simulink model "Problema_2_simulink_f"  (R2014a)
settings: Solver=ode45  StartTime=0.0  StopTime=10  RelTol=1e-3
values from neighbouring files (symbols this model uses):
  b = 0.5    [Problema_2_tp2_variables.m]
  Feq = (k * ieq^2)/yeq    (= 1.96001568013)    [Problema_2_tp2_variables.m]
  g = 9.8    [Problema_2_tp2_variables.m]
  ieq = 0.5    [Problema_2_tp2_variables.m]
  ki = (2 * ieq * k)/yeq    (= 7.8400627205)    [Problema_2_tp2_variables.m]
  ky = -(k * ieq^2)/yeq^2    (= -7.68332293268)    [Problema_2_tp2_variables.m]
  L = 0.01    [Problema_2_tp2_variables.m]
  M = 0.2    [Problema_2_tp2_variables.m]
  R = 20    [Problema_2_tp2_variables.m]
  yeq = 0.2551    [Problema_2_tp2_variables.m]
undefined symbols (not defined in the file or in its folder): bs, s
settings Model: Creator=lraff  LastModifiedBy=lraff
settings DataIOCC: LimitDataPoints=off  MaxDataPoints=5000

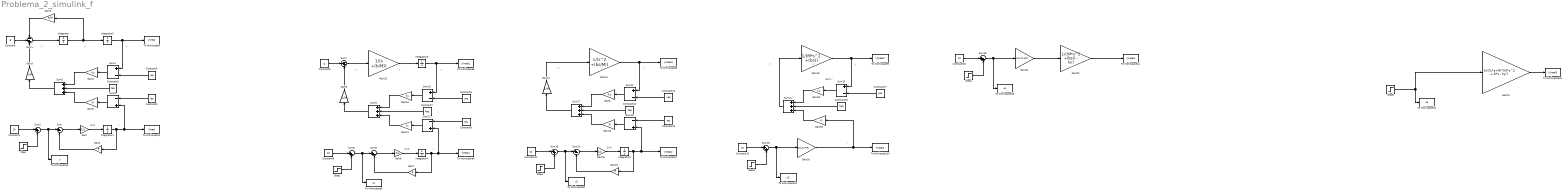
== system Problema_2_simulink_f ==
  note: di/dt
  note: i
  note: y''
  note: y'
  note: y
  note: di/dt
  note: i
  note: y''
  note: y'
  note: y
  note: di/dt
  note: i
  note: y''
  note: y'
  note: y
  note: i
  note: y''
  note: y'
  note: y
  note: delta y
  Constant : Constant  Value=g
  Constant{1,6,10..11,16} (5 alike) : Constant  Value=10
  Constant{2,7,12,15} (4 alike) : Constant  Value=Feq
  Constant13 : Constant  Value=ieq
  Constant{4,9,14,17} (4 alike) : Constant  Value=yeq
  Constant3 : Constant  Value=ieq
  Constant5 : Constant  Value=g
  Constant8 : Constant  Value=ieq
  Gain : Gain  Gain=1/L
  Gain1 : Gain  Gain=R
  Gain{4,8,10,23} (4 alike) : Gain  Gain=ky
  Gain{5,11,13,18} (4 alike) : Gain  Gain=ki
  Gain12 : Gain  Gain=1/(s +(b/M))
  Gain14 : Gain  Gain=1/(s^2 +(bs/M))
  Gain15 : Gain  Gain=1/L
  Gain16 : Gain  Gain=R
  Gain17 : Gain  Gain=1/M
  Gain19 : Gain  Gain=1/(M*s^2 +(bs))
  Gain2 : Gain  Gain=b/M
  Gain20 : Gain  Gain=1/(L*s+R)
  Gain21 : Gain  Gain=ki/((L*s+R)*(M*s^2 + b*s - ky))
  Gain22 : Gain  Gain=1/((M*s^2 +(bs)) - ky)
  Gain24 : Gain  Gain=ki/(L*s+R)
  Gain3 : Gain  Gain=1/M
  Gain6 : Gain  Gain=1/L
  Gain7 : Gain  Gain=R
  Gain9 : Gain  Gain=1/M
  Integrator : Integrator
  Integrator1 : Integrator  InitialCondition=0.5
  Integrator2 : Integrator  InitialCondition=0.2551
  Integrator3 : Integrator  InitialCondition=0.5
  Integrator4 : Integrator  InitialCondition=0.5
  Integrator5 : Integrator  InitialCondition=0.2551
  Step{,1..5} (6 alike) : Step  After=0.2  SampleTime=0
  Sum : Sum  Inputs=|+-
  Sum1 : Sum  Inputs=--+
  Sum{4,10,12,15} (4 alike) : Sum  Inputs=+-
  Sum11 : Sum  Inputs=-+
  Sum13 : Sum  Inputs=-+
  Sum14 : Sum  Inputs=|+-
  Sum{2,8,16,19..20} (5 alike) : Sum  Inputs=|++
  Sum{3,9,17,21} (4 alike) : Sum  Inputs=+++
  Sum5 : Sum  Inputs=-+
  Sum6 : Sum  Inputs=|+-
  Sum7 : Sum  Inputs=--+
  To Workspace : ToWorkspace  VariableName=ylineal  SaveFormat=Timeseries  SampleTime=-1
  To Workspace1 : ToWorkspace  VariableName=ilineal  SaveFormat=Timeseries  SampleTime=-1
  To Workspace10 : ToWorkspace  VariableName=ilineal3  SaveFormat=Timeseries  SampleTime=-1
  To Workspace11 : ToWorkspace  VariableName=u3  SaveFormat=Timeseries  SampleTime=-1
  To Workspace12 : ToWorkspace  VariableName=u5  SaveFormat=Timeseries  SampleTime=-1
  To Workspace13 : ToWorkspace  VariableName=u4  SaveFormat=Timeseries  SampleTime=-1
  To Workspace14 : ToWorkspace  VariableName=ylineal4  SaveFormat=Timeseries  SampleTime=-1
  To Workspace15 : ToWorkspace  VariableName=ylineal5  SaveFormat=Timeseries  SampleTime=-1
  To Workspace2 : ToWorkspace  VariableName=u  SaveFormat=Timeseries  SampleTime=-1
  To Workspace3 : ToWorkspace  VariableName=ylineal1  SaveFormat=Timeseries  SampleTime=-1
  To Workspace4 : ToWorkspace  VariableName=ilineal1  SaveFormat=Timeseries  SampleTime=-1
  To Workspace5 : ToWorkspace  VariableName=u1  SaveFormat=Timeseries  SampleTime=-1
  To Workspace6 : ToWorkspace  VariableName=ylineal2  SaveFormat=Timeseries  SampleTime=-1
  To Workspace7 : ToWorkspace  VariableName=ilineal2  SaveFormat=Timeseries  SampleTime=-1
  To Workspace8 : ToWorkspace  VariableName=u2  SaveFormat=Timeseries  SampleTime=-1
  To Workspace9 : ToWorkspace  VariableName=ylineal3  SaveFormat=Timeseries  SampleTime=-1
  wires:
  Sum/1 -> Gain/1
  Gain/1 -> Integrator1/1
  Gain1/1 -> Sum/2
  Integrator1/1 -> Sum5/2, To Workspace1/1, Gain1/1
  Sum1/1 -> Integrator/1
  Integrator/1 -> Gain2/1, Integrator2/1
  Gain2/1 -> Sum1/1
  Integrator2/1 -> To Workspace/1, Sum4/1
  Constant/1 -> Sum1/2
  Constant1/1 -> Sum2/1
  Sum2/1 -> To Workspace2/1, Sum/1
  Constant2/1 -> Sum3/2
  Constant4/1 -> Sum4/2
  Constant3/1 -> Sum5/1
  Sum4/1 -> Gain4/1
  Gain4/1 -> Sum3/1
  Sum5/1 -> Gain5/1
  Gain5/1 -> Sum3/3
  Sum3/1 -> Gain3/1
  Gain3/1 -> Sum1/3
  Step/1 -> Sum2/2
  Sum6/1 -> Gain6/1
  Gain6/1 -> Integrator4/1
  Gain7/1 -> Sum6/2
  Integrator4/1 -> Sum11/2, To Workspace4/1, Gain7/1
  Sum7/1 -> Gain12/1
  Gain12/1 -> Integrator5/1
  Integrator5/1 -> To Workspace3/1, Sum10/1
  Constant5/1 -> Sum7/2
  Constant6/1 -> Sum8/1
  Sum8/1 -> To Workspace5/1, Sum6/1
  Constant7/1 -> Sum9/2
  Constant9/1 -> Sum10/2
  Constant8/1 -> Sum11/1
  Sum10/1 -> Gain10/1
  Gain10/1 -> Sum9/1
  Sum11/1 -> Gain11/1
  Gain11/1 -> Sum9/3
  Sum9/1 -> Gain9/1
  Gain9/1 -> Sum7/3
  Step1/1 -> Sum8/2
  Sum14/1 -> Gain15/1
  Gain15/1 -> Integrator3/1
  Gain16/1 -> Sum14/2
  Integrator3/1 -> Sum13/2, To Workspace7/1, Gain16/1
  Gain17/1 -> Gain14/1
  Gain14/1 -> Sum12/1, To Workspace6/1
  Constant11/1 -> Sum16/1
  Sum16/1 -> To Workspace8/1, Sum14/1
  Constant12/1 -> Sum17/2
  Constant14/1 -> Sum12/2
  Constant13/1 -> Sum13/1
  Sum12/1 -> Gain8/1
  Gain8/1 -> Sum17/1
  Sum13/1 -> Gain13/1
  Gain13/1 -> Sum17/3
  Sum17/1 -> Gain17/1
  Step2/1 -> Sum16/2
  Sum20/1 -> Gain20/1, To Workspace11/1
  Sum21/1 -> Gain19/1
  Gain19/1 -> Sum15/1, To Workspace9/1
  Constant10/1 -> Sum20/1
  Constant15/1 -> Sum21/2
  Constant17/1 -> Sum15/2
  Sum15/1 -> Gain23/1
  Gain23/1 -> Sum21/1
  Gain20/1 -> Gain18/1, To Workspace10/1
  Gain18/1 -> Sum21/3
  Step3/1 -> Sum20/2
  Sum19/1 -> Gain24/1, To Workspace13/1
  Gain24/1 -> Gain22/1
  Constant16/1 -> Sum19/1
  Gain22/1 -> To Workspace14/1
  Step4/1 -> Sum19/2
  Step5/1 -> Gain21/1, To Workspace12/1
  Gain21/1 -> To Workspace15/1
